simulink library "PubLib"  (R2020b)
settings: Solver=VariableStepAuto  StartTime=0.0  StopTime=10.0  RelTol=1e-3
settings Model: Creator=GW00166368  LastModifiedBy=GW00166368

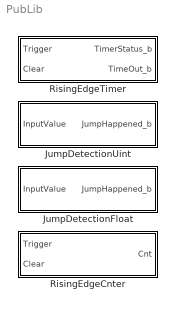
== system PubLib ==
  JumpDetectionFloat : Subsystem  mask(JumpDetectionFloat){StartValue=0, FinishValue=0, Tolerance=0}
      mask help: 检测一个周期内，浮点数输入是否存在从StartValue到FinishValue的跳变，允许Tolerance的误差
  JumpDetectionUint : Subsystem  mask(JumpDetectionUint){StartValue=0, FinishValue=0}
      mask help: 检测一个周期内，整形输入是否存在从StartValue到FinishValue的跳变，StartValue和FinishValue非整数时四舍五入取整。
  RisingEdgeCnter : Subsystem  mask(RisingEdgeCnter){}
      mask help: 每当rigger（Boolean）端口检测到一次上升沿后，计数一次。当Clear（Boolean）端口检测到true后，计数器清零。输出计数次数
  RisingEdgeTimer : Subsystem  mask(RisingEdgeTimer){MaxCnt=0}
      mask help: 当Trigger（Boolean）端口检测到上升沿后，开始计数，输出TimerStatus_b（Boolean）为true。当计数达到MaxCnt时，或Clear（Boolean）端口检测到true后，计数器清零。TimerStatus_b输出false。若MaxCycles==0，则只能由Clear端口输入true将输出置false。

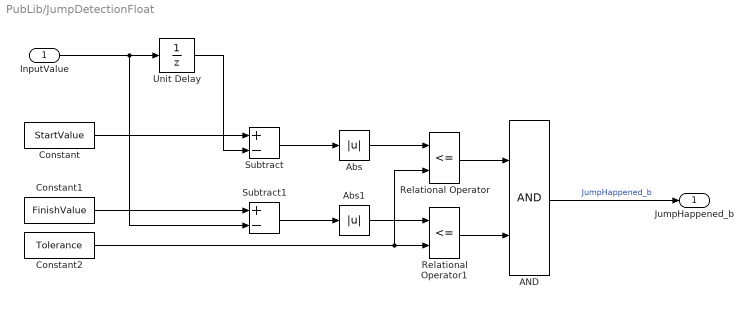
== system PubLib/JumpDetectionFloat ==
  InputValue : Inport  OutDataTypeStr=single
  AND : Logic  AllPortsSameDT=off  OutDataTypeStr=boolean
  Abs : Abs
  Abs1 : Abs
  Constant : Constant  Value=StartValue  OutDataTypeStr=single
  Constant1 : Constant  Value=FinishValue  OutDataTypeStr=single
  Constant2 : Constant  Value=Tolerance  OutDataTypeStr=single
  Relational Operator : RelationalOperator  Operator=<=  OutDataTypeStr=boolean  RndMeth=Simplest
  Relational Operator1 : RelationalOperator  Operator=<=  OutDataTypeStr=boolean  RndMeth=Simplest
  Subtract : Sum  Inputs=+-
  Subtract1 : Sum  Inputs=+-
  Unit Delay : UnitDelay  SampleTime=-1  HasFrameUpgradeWarning=on
  JumpHappened_b : Outport
  wires:
  Unit Delay/1 -> Subtract/2
  Constant1/1 -> Subtract1/1
  Subtract1/1 -> Abs1/1
  Abs1/1 -> Relational Operator1/1
  Constant2/1 -> Relational Operator/2, Relational Operator1/2
  Abs/1 -> Relational Operator/1
  Subtract/1 -> Abs/1
  Constant/1 -> Subtract/1
  InputValue/1 -> Unit Delay/1, Subtract1/2
  Relational Operator/1 -> AND/1
  Relational Operator1/1 -> AND/2
  AND/1 -> JumpHappened_b/1  "JumpHappened_b"

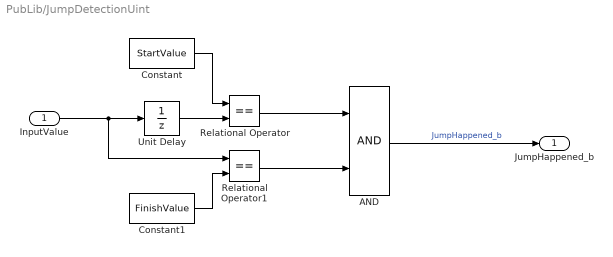
== system PubLib/JumpDetectionUint ==
  InputValue : Inport  OutDataTypeStr=uint8
  AND : Logic  AllPortsSameDT=off  OutDataTypeStr=boolean
  Constant : Constant  Value=StartValue  OutDataTypeStr=uint8
  Constant1 : Constant  Value=FinishValue  OutDataTypeStr=uint8
  Relational Operator : RelationalOperator  Operator===  OutDataTypeStr=boolean  RndMeth=Simplest
  Relational Operator1 : RelationalOperator  Operator===  OutDataTypeStr=boolean  RndMeth=Simplest
  Unit Delay : UnitDelay  SampleTime=-1  HasFrameUpgradeWarning=on
  JumpHappened_b : Outport
  wires:
  Constant1/1 -> Relational Operator1/2
  Constant/1 -> Relational Operator/1
  AND/1 -> JumpHappened_b/1  "JumpHappened_b"
  Relational Operator1/1 -> AND/2
  Relational Operator/1 -> AND/1
  InputValue/1 -> Unit Delay/1, Relational Operator1/1
  Unit Delay/1 -> Relational Operator/2

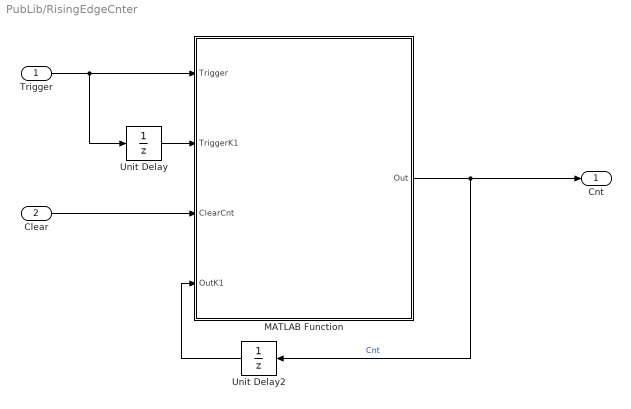
== system PubLib/RisingEdgeCnter ==
  Trigger : Inport  OutDataTypeStr=boolean
  Clear : Inport  Port=2  OutDataTypeStr=boolean
  MATLAB Function : MATLAB Function  TreatAsAtomicUnit=on
  Unit Delay : UnitDelay  SampleTime=-1  HasFrameUpgradeWarning=on
  Unit Delay2 : UnitDelay  SampleTime=-1  HasFrameUpgradeWarning=on
  Cnt : Outport  OutDataTypeStr=uint8
  wires:
  Clear/1 -> MATLAB Function/3(ClearCnt)
  Trigger/1 -> MATLAB Function/1(Trigger), Unit Delay/1
  Unit Delay/1 -> MATLAB Function/2(TriggerK1)
  MATLAB Function/1(Out) -> Cnt/1, Unit Delay2/1  "Cnt"
  Unit Delay2/1 -> MATLAB Function/4(OutK1)

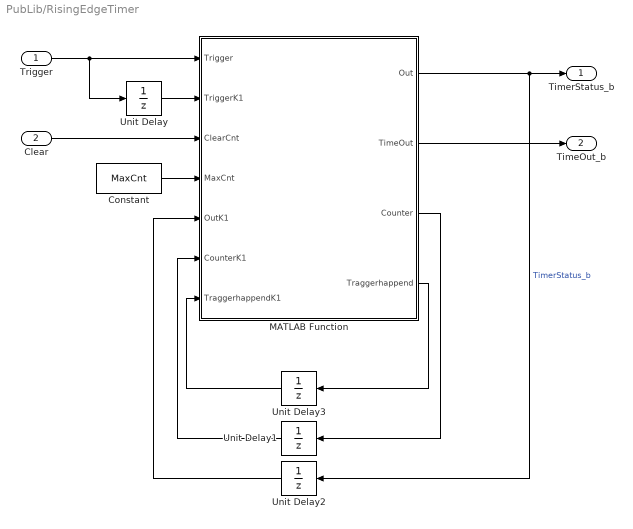
== system PubLib/RisingEdgeTimer ==
  Trigger : Inport  OutDataTypeStr=boolean
  Clear : Inport  Port=2  OutDataTypeStr=boolean
  Constant : Constant  Value=MaxCnt  OutDataTypeStr=uint16
  MATLAB Function : MATLAB Function  TreatAsAtomicUnit=on
  Unit Delay{,1..3} (4 alike) : UnitDelay  SampleTime=-1  HasFrameUpgradeWarning=on
  TimerStatus_b : Outport  OutDataTypeStr=boolean
  TimeOut_b : Outport  Port=2  OutDataTypeStr=boolean
  wires:
  Unit Delay2/1 -> MATLAB Function/5(OutK1)
  MATLAB Function/1(Out) -> Unit Delay2/1, TimerStatus_b/1  "TimerStatus_b"
  Constant/1 -> MATLAB Function/4(MaxCnt)
  MATLAB Function/3(Counter) -> Unit Delay1/1
  Unit Delay/1 -> MATLAB Function/2(TriggerK1)
  Unit Delay1/1 -> MATLAB Function/6(CounterK1)
  Trigger/1 -> MATLAB Function/1(Trigger), Unit Delay/1
  Clear/1 -> MATLAB Function/3(ClearCnt)
  MATLAB Function/2(TimeOut) -> TimeOut_b/1
  MATLAB Function/4(Traggerhappend) -> Unit Delay3/1
  Unit Delay3/1 -> MATLAB Function/7(TraggerhappendK1)

== matlab function PubLib/RisingEdgeTimer/MATLAB Function ==
  data: Trigger input boolean; Out output boolean; TimeOut output boolean; TriggerK1 input boolean; ClearCnt input boolean; MaxCnt input uint16; OutK1 input boolean; CounterK1 input uint16; Counter output uint16; TraggerhappendK1 input boolean; Traggerhappend output boolean
function [Out,TimeOut,Counter,Traggerhappend] = RisingEdgeTimer(Trigger,TriggerK1, ClearCnt, MaxCnt,OutK1, CounterK1,TraggerhappendK1)
%#codegen
TimeOut=false;
Traggerhappend=TraggerhappendK1;
if MaxCnt~=0
    if (Trigger==1)&&(TriggerK1==0)
        Counter = MaxCnt;
        Traggerhappend=true;
    elseif CounterK1 > 0x0
        Counter = CounterK1 - uint16(1);
    else
        Counter = CounterK1;
    end 
    if ClearCnt
        Traggerhappend=false;
        Counter = uint16(0);
    end
    if Counter > 0x0
        Out = true;
    else
        Out = false;
    end
else
    Counter = uint16(0);
    if (Trigger==1)&&(TriggerK1==0)
        Out=true;
    else
        Out=OutK1;
    end
    if ClearCnt
        Out=false;
    end
end
if Counter==uint16(0) && Trigger==1 && Traggerhappend
    TimeOut=true;
end 
if Trigger==0
    Traggerhappend=false;
end
end

== matlab function PubLib/RisingEdgeCnter/MATLAB Function ==
  data: Trigger input boolean; Out output uint8; TriggerK1 input boolean; ClearCnt input boolean; OutK1 input uint8
function Out  = RisingEdgeTimer(Trigger,TriggerK1, ClearCnt, OutK1)
%#codegen
    if (Trigger==1)&&(TriggerK1==0)
        Out = OutK1+1;     
    else
        Out = OutK1;
    end 
    if ClearCnt
        Out = uint8(0);
    end
end
